simulink model "fermentation_simple_model"  (R2017b)
settings: Solver=VariableStepAuto  StartTime=0.0  StopTime=250  RelTol=1e-3
values from neighbouring files (symbols this model uses):
  E_0 = 0    [fermentation_config.m]    (also in fermentation_config_update.m)
  G_0 = 70    [fermentation_config.m]    (also in fermentation_config_update.m = 104.992339972)
  M_0 = 40    [fermentation_config.m]    (also in fermentation_config_update.m = 60)
  N_0 = 230    [fermentation_config.m]    (also in fermentation_config_update.m = 343.376857703)
  R_EG = 1.92    [fermentation_config.m]    (also in fermentation_config_update.m)
  R_EM = 3.84    [fermentation_config.m]    (also in fermentation_config_update.m)
  R_EN = 5.76    [fermentation_config.m]    (also in fermentation_config_update.m)
  R_XG = 0.134    [fermentation_config.m]    (also in fermentation_config_update.m)
  R_XM = 0.268    [fermentation_config.m]    (also in fermentation_config_update.m)
  R_XN = 0.402    [fermentation_config.m]    (also in fermentation_config_update.m)
  X_0 = 200    [fermentation_config.m]    (also in fermentation_config_update.m)
settings Model: PauseTimes=0  Creator=Oscar  LastModifiedBy=Oscar

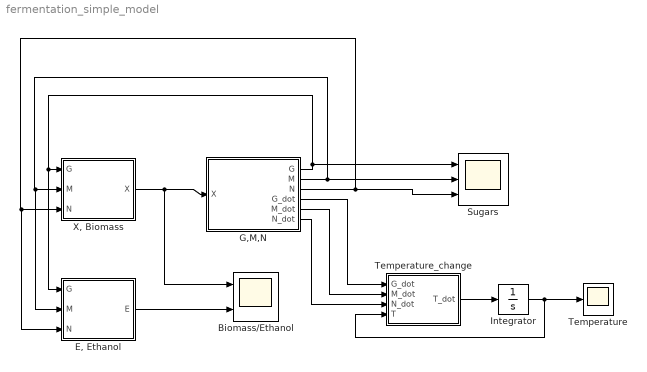
== system fermentation_simple_model ==
  Biomass/Ethanol : Scope  NumInputPorts=2
  "E, Ethanol" : Subsystem
  G,M,N : Subsystem
  Integrator : Integrator  InitialCondition=10
  Sugars : Scope  NumInputPorts=3
  Temperature : Scope
  Temperature_change : MATLAB Function  TreatAsAtomicUnit=on
  "X, Biomass " : Subsystem
  wires:
  "X, Biomass "/1(X) -> Biomass/Ethanol/1, G,M,N/1(X)
  G,M,N/1(G) -> "E, Ethanol"/1(G), "X, Biomass "/1(G), Sugars/1
  G,M,N/2(M) -> Sugars/2, "E, Ethanol"/2(M), "X, Biomass "/2(M)
  G,M,N/3(N) -> Sugars/3, "E, Ethanol"/3(N), "X, Biomass "/3(N)
  "E, Ethanol"/1(E) -> Biomass/Ethanol/2
  G,M,N/4(G_dot) -> Temperature_change/1(G_dot)
  G,M,N/5(M_dot) -> Temperature_change/2(M_dot)
  G,M,N/6(N_dot) -> Temperature_change/3(N_dot)
  Temperature_change/1(T_dot) -> Integrator/1
  Integrator/1 -> Temperature_change/4(T), Temperature/1

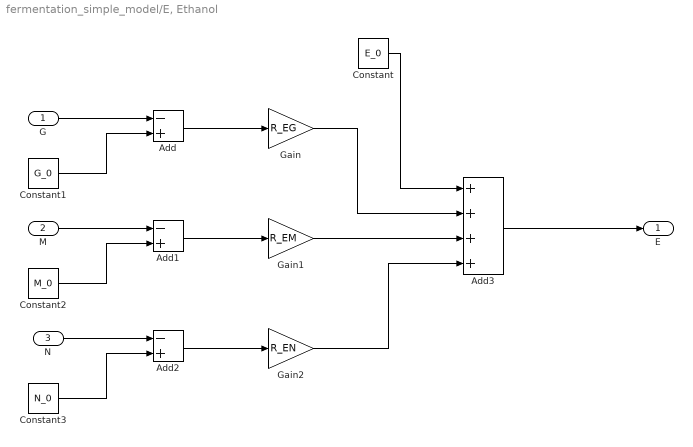
== system fermentation_simple_model/E, Ethanol ==
  G : Inport
  M : Inport  Port=2
  N : Inport  Port=3
  Add : Sum  Inputs=-+
  Add1 : Sum  Inputs=-+
  Add2 : Sum  Inputs=-+
  Add3 : Sum  Inputs=++++
  Constant : Constant  Value=E_0
  Constant1 : Constant  Value=G_0
  Constant2 : Constant  Value=M_0
  Constant3 : Constant  Value=N_0
  Gain : Gain  Gain=R_EG
  Gain1 : Gain  Gain=R_EM
  Gain2 : Gain  Gain=R_EN
  E : Outport
  wires:
  G/1 -> Add/1
  M/1 -> Add1/1
  N/1 -> Add2/1
  Constant3/1 -> Add2/2
  Constant2/1 -> Add1/2
  Constant1/1 -> Add/2
  Add/1 -> Gain/1
  Add1/1 -> Gain1/1
  Add2/1 -> Gain2/1
  Add3/1 -> E/1
  Constant/1 -> Add3/1
  Gain/1 -> Add3/2
  Gain1/1 -> Add3/3
  Gain2/1 -> Add3/4

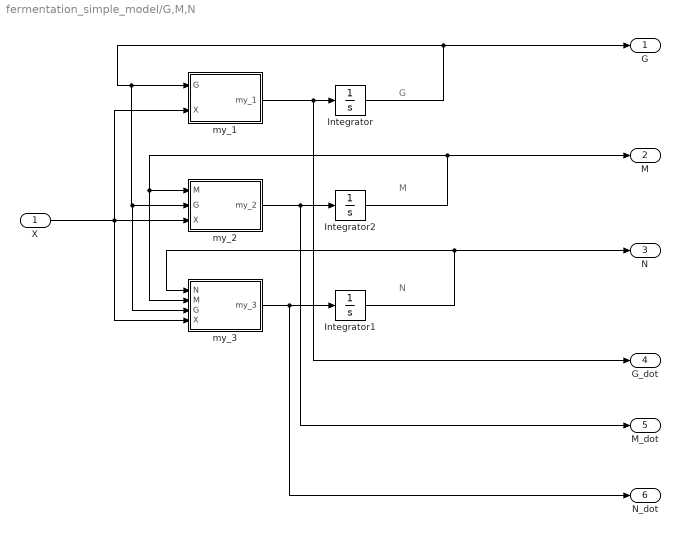
== system fermentation_simple_model/G,M,N ==
  note: N
  note: M
  note: G
  X : Inport
  Integrator : Integrator  InitialCondition=G_0
  Integrator1 : Integrator  InitialCondition=N_0
  Integrator2 : Integrator  InitialCondition=M_0
  my_1 : MATLAB Function  TreatAsAtomicUnit=on
  my_2 : MATLAB Function  TreatAsAtomicUnit=on
  my_3 : MATLAB Function  TreatAsAtomicUnit=on
  G : Outport
  M : Outport  Port=2
  N : Outport  Port=3
  G_dot : Outport  Port=4
  M_dot : Outport  Port=5
  N_dot : Outport  Port=6
  wires:
  X/1 -> my_1/2(X), my_2/3(X), my_3/4(X)
  my_1/1(my_1) -> G_dot/1, Integrator/1
  Integrator/1 -> G/1, my_1/1(G), my_3/3(G), my_2/2(G)
  my_2/1(my_2) -> M_dot/1, Integrator2/1
  Integrator1/1 -> my_3/1(N), N/1
  Integrator2/1 -> my_3/2(M), my_2/1(M), M/1
  my_3/1(my_3) -> N_dot/1, Integrator1/1

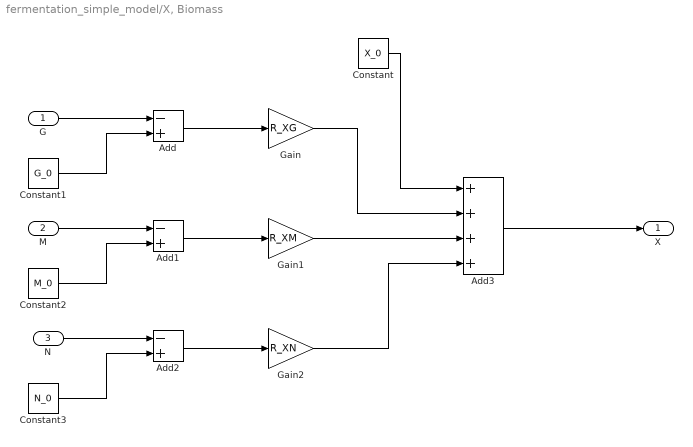
== system fermentation_simple_model/X, Biomass  ==
  G : Inport
  M : Inport  Port=2
  N : Inport  Port=3
  Add : Sum  Inputs=-+
  Add1 : Sum  Inputs=-+
  Add2 : Sum  Inputs=-+
  Add3 : Sum  Inputs=++++
  Constant : Constant  Value=X_0
  Constant1 : Constant  Value=G_0
  Constant2 : Constant  Value=M_0
  Constant3 : Constant  Value=N_0
  Gain : Gain  Gain=R_XG
  Gain1 : Gain  Gain=R_XM
  Gain2 : Gain  Gain=R_XN
  X : Outport
  wires:
  G/1 -> Add/1
  M/1 -> Add1/1
  N/1 -> Add2/1
  Constant3/1 -> Add2/2
  Constant2/1 -> Add1/2
  Constant1/1 -> Add/2
  Add/1 -> Gain/1
  Add1/1 -> Gain1/1
  Add2/1 -> Gain2/1
  Add3/1 -> X/1
  Constant/1 -> Add3/1
  Gain/1 -> Add3/2
  Gain1/1 -> Add3/3
  Gain2/1 -> Add3/4

== matlab function fermentation_simple_model/G,M,N/my_2 ==
  data: M input; G input; my_2 output; X input
function my_2 = fcn(M,G,X)
%#codegen
i = 2;
% maximum reaction velocity for ith sugar (G, M, N), h^-1
V_M = [0.0144, 0.0268, 0.028, 0.0364]';
% Michaelis constant for ith sugar  (G, M, N), mol/m^3
K_M = [1100, 814, 610, 360]';
% inhibition constant for ith sugar (G, M)
Ki_G = [123, 182, 240, 262]';

my_2 = -((V_M(i)*M)/(K_M(i) + M)*(Ki_G(i)/(Ki_G(i) + G)))*X;

== matlab function fermentation_simple_model/G,M,N/my_1 ==
  data: G input; my_1 output; X input
function my_1 = fcn(G,X)
%#codegen
i = 2;
% maximum reaction velocity for ith sugar (G, M, N), h^-1
V_G = [0.0048, 0.013, 0.015, 0.0302]';
% Michaelis constant for ith sugar  (G, M, N), mol/m^3
K_G = [23.5, 4.7, 1.8, 0.102]';

my_1 = -(V_G(i)*G)/(K_G(i) + G)*X;

== matlab function fermentation_simple_model/G,M,N/my_3 ==
  data: N input; M input; G input; my_3 output; X input
function my_3 = fcn(N,M,G,X)
%#codegen
i = 2;
% maximum reaction velocity for ith sugar (G, M, N), h^-1
V_N = [0.087, 0.113, 0.13, 0.151]';
% Michaelis constant for ith sugar  (G, M, N), mol/m^3
K_N = [10900, 7160, 4460, 2410]';
% inhibition constant for ith sugar (G, M)
Ki_G = [123, 182, 240, 262]';
Ki_M = [2090, 6360, 8010, 17500]';


my_3 = -((V_N(i)*N)/(K_N(i) + N)*Ki_M(i)/(Ki_M(i) + M)*Ki_G(i)/(Ki_G(i) + G))*X;

== matlab function fermentation_simple_model/Temperature_change ==
  data: G_dot input; T_dot output; M_dot input; N_dot input; T input
function T_dot = fcn(G_dot,M_dot,N_dot,T)
%#codegen

rho = 1.06;
Cp = 4000;

DH_RG = -91.2;
DH_RM = -226.3;
DH_RN = -361.3;

% coolant temperature
T_c = 10;

U = 1300;
Area = 0.188;
V = 1;

u = (U*Area)/V;

T_dot = 1/(rho*Cp)*(DH_RG*G_dot + DH_RM*M_dot + DH_RN*N_dot - u*(T - T_c));
